simulink model "oscillatorSimulink"  (Simulink 10.1)
settings: Solver=VariableStepAuto  StartTime=0.0  StopTime=20.0  RelTol=1e-3
values from neighbouring files (symbols this model uses):
  C = 0.25    [constants1.m]    (also in oscillator.m)
  L = 1.6    [constants1.m]    (also in oscillator.m)
  R1 = 4    [constants1.m]    (also in oscillator.m)
  R2 = 2    [constants1.m]    (also in oscillator.m)
  R3 = 3    [constants1.m]    (also in oscillator.m)
settings Model: Creator=M. Tilocca  LastModifiedBy=M. Tilocca
settings DataIOCC: SaveFormat=Dataset  ReturnWorkspaceOutputs=on
settings OptimizationCC: LifeSpan=auto
settings DebuggingCC: UnderspecifiedInitializationDetection=Simplified  MergeDetectMultiDrivingBlocksExec=error  SFUnexpectedBacktrackingDiag=error  SFNoUnconditionalDefaultTransitionDiag=error  SFExecutionAtInitializationDiag=warning  ArithmeticOperatorsInVariantConditions=error
settings HardwareCC: ProdBitPerPointer=64  ProdBitPerSizeT=64  ProdBitPerPtrDiffT=64  ProdLargestAtomicFloat=Float  ProdIntDivRoundTo=Zero  ProdEndianess=LittleEndian  ProdWordSize=64  ProdHWDeviceType=Intel->x86-64 (Windows64)
settings ModelReferenceCC: PropagateSignalLabelsOutOfModel=on
settings SFSimCC: SimUseLocalCustomCode=on  CustomCodeUndefinedFunction=FilterOut
settings RTWCC: RTWUseLocalCustomCode=on
settings CodeAppCC: StateflowObjectComments=off
settings GRTTargetCC: TargetLangStandard=C99 (ISO)  CombineOutputUpdateFcns=on  GRTInterface=off
settings ConfigComp: CovMetricSettings=dwe  CovHtmlReporting=off  CovSaveCumulativeToWorkspaceVar=off  CovSaveSingleToWorkspaceVar=off  CovExternalEMLEnable=on

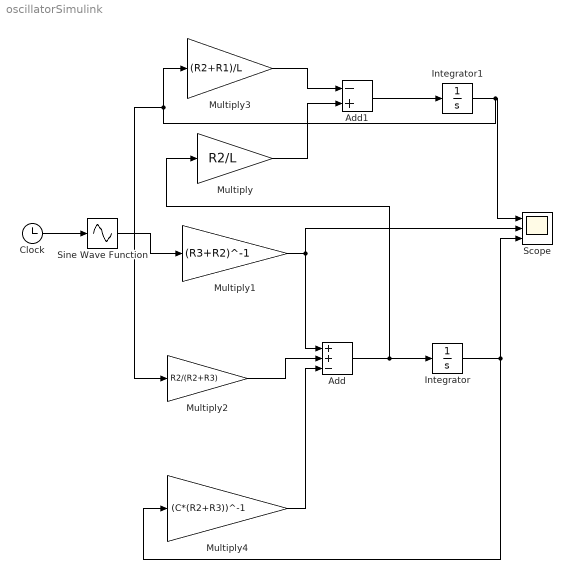
== system oscillatorSimulink ==
  Add : Sum  Inputs=++-
  Add1 : Sum  Inputs=-+
  Clock : Clock
  Integrator : Integrator  InitialCondition=2
  Integrator1 : Integrator  InitialCondition=15
  Multiply : Gain  Gain=R2/L
  Multiply1 : Gain  Gain=(R3+R2)^-1
  Multiply2 : Gain  Gain=R2/(R2+R3)
  Multiply3 : Gain  Gain=(R2+R1)/L
  Multiply4 : Gain  Gain=(C*(R2+R3))^-1
  Scope : Scope  NumInputPorts=3
  Sine Wave Function : Sin  TimeSource=Use external signal  SampleTime=0
  wires:
  Clock/1 -> Sine Wave Function/1
  Sine Wave Function/1 -> Multiply1/1
  Multiply3/1 -> Add1/1
  Add1/1 -> Integrator1/1
  Multiply/1 -> Add1/2
  Multiply1/1 -> Add/1, Scope/2
  Multiply2/1 -> Add/2
  Multiply4/1 -> Add/3
  Add/1 -> Multiply/1, Integrator/1
  Integrator/1 -> Multiply4/1, Scope/3
  Integrator1/1 -> Multiply2/1, Multiply3/1, Scope/1
